simulink model "M004_refor_control"  (R2021a)
settings: Solver=VariableStepAuto  StartTime=0.0  StopTime=3  RelTol=1e-3
values from neighbouring files (symbols this model uses):
  MM = struct2array(MM)    [M004_init_refor_meca.m]
undefined symbols (not defined in the file or in its folder): params
settings Model: Creator=djoroya  LastModifiedBy=djoroya

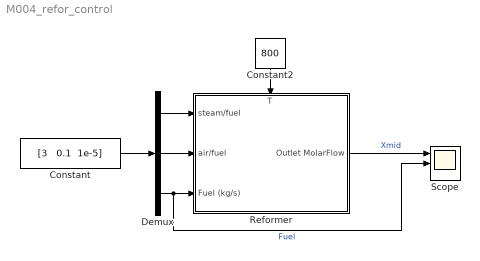
== system M004_refor_control ==
  Constant : Constant  Value="[3   0.1  1e-5]"
  Constant2 : Constant  Value=800
  Demux : Demux  Outputs=3
  Reformer : Subsystem
      settings: PortSchema="{\"entries\":[{\"content\":{\"sides\":[{\"content\":{\"connectorIds\":[\"In1\",\"In2\",\"In3\"]},\"type\":\"ConnectorPlacement.EquallySpacedRectSide\",\"uuid\":\"bba98e9a-4a8f-433d-80b6-6443373beb37\"},{\"content\":{\"connectorIds\":[\"Out1\"],\"side\":\"RIGHT\"},\"type\":\"ConnectorPlacement.EquallySpacedRectSide\",\"uuid\":\"bb8208fa-3ad6-4550-bb87-9c458da504c5\"},{\"content\":{\"connectorIds\":[\"In4\"],\"side\":\"TOP\"},\"type\":\"ConnectorPlacement.EquallySpacedRectSide\",\"uuid\":\"10760c79-2681-4834-b090-bc5e1ffe83d8\"}]},\"type\":\"ConnectorPlacement.EquallySpacedConnector\",\"uuid\":\"c7bbf7d3-64d5-4f0e-88ff-bb50ba74e7ab\"}],\"packageUris\":[\"http://schema.mathworks.com/mf0/Connector/R2020b\"],\"version\":\"1.0\"}"
  Scope : Scope  NumInputPorts=3
  wires:
  Reformer/1(Outlet MolarFlow) -> Scope/1  "Xmid"
  Constant2/1 -> Reformer/4(T)
  Constant/1 -> Demux/1
  Demux/2 -> Reformer/2(air/fuel)
  Demux/3 -> Scope/2, Reformer/3(Fuel (kg/s))  "Fuel"
  Demux/1 -> Reformer/1(steam/fuel)

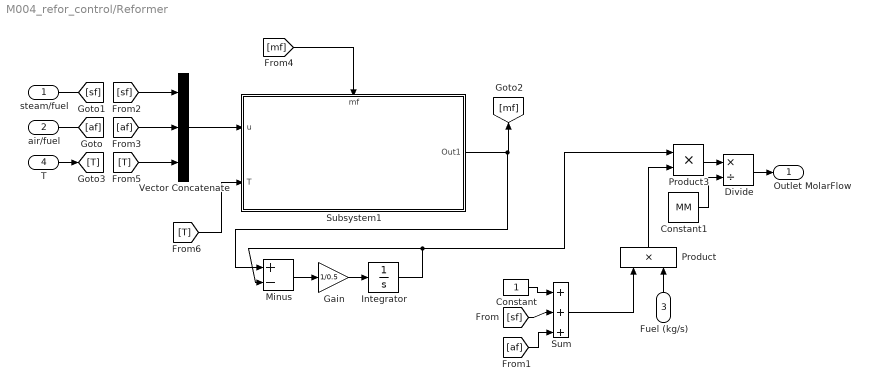
== system M004_refor_control/Reformer ==
  steam/fuel : Inport
  air/fuel : Inport  Port=2
  Fuel (kg/s) : Inport  Port=3
  T : Inport  Port=4
  Constant : Constant
  Constant1 : Constant  Value=MM
  Divide : Product  Inputs=*/
  Gain : Gain  Gain=1/0.5
  Integrator : Integrator
  Minus : Sum  Inputs=+-
  Product : Product
  Product3 : Product
  Subsystem1 : Subsystem
      settings: PortSchema="{\"entries\":[{\"content\":{\"sides\":[{\"content\":{\"connectorIds\":[\"In1\",\"In2\"]},\"type\":\"ConnectorPlacement.EquallySpacedRectSide\",\"uuid\":\"d4e99106-98ee-451f-9de6-7a659962116b\"},{\"content\":{\"connectorIds\":[\"Out1\"],\"side\":\"RIGHT\"},\"type\":\"ConnectorPlacement.EquallySpacedRectSide\",\"uuid\":\"1c23e47e-8482-4a31-825f-a97525afd909\"},{\"content\":{\"connectorIds\":[\"In3\"],\"side\":\"TOP\"},\"type\":\"ConnectorPlacement.EquallySpacedRectSide\",\"uuid\":\"6970ef93-3b6d-46bc-9d04-0338d9ef962f\"}]},\"type\":\"ConnectorPlacement.EquallySpacedConnector\",\"uuid\":\"3dd46f6e-571c-473b-b07f-3e0a0086d241\"}],\"packageUris\":[\"http://schema.mathworks.com/mf0/Connector/R2020b\"],\"version\":\"1.0\"}"
  Sum : Sum  Inputs=|+++
  Vector Concatenate : Concatenate  NumInputs=3
  Outlet MolarFlow : Outport
  wires:
  [af] -> Vector Concatenate/2
  [sf] -> Vector Concatenate/1
  [sf] -> Sum/2
  steam/fuel/1 -> [sf]
  Product/1 -> Product3/2
  air/fuel/1 -> [af]
  [af] -> Sum/3
  Constant/1 -> Sum/1
  Fuel (kg/s)/1 -> Product/2
  Sum/1 -> Product/1
  T/1 -> [T]
  [T] -> Vector Concatenate/3
  Subsystem1/1(Out1) -> [mf], Minus/1
  Vector Concatenate/1 -> Subsystem1/1(u)
  [mf] -> Subsystem1/3(mf)
  [T] -> Subsystem1/2(T)
  Integrator/1 -> Product3/1, Minus/2
  Minus/1 -> Gain/1
  Gain/1 -> Integrator/1
  Product3/1 -> Divide/1
  Divide/1 -> Outlet MolarFlow/1
  Constant1/1 -> Divide/2

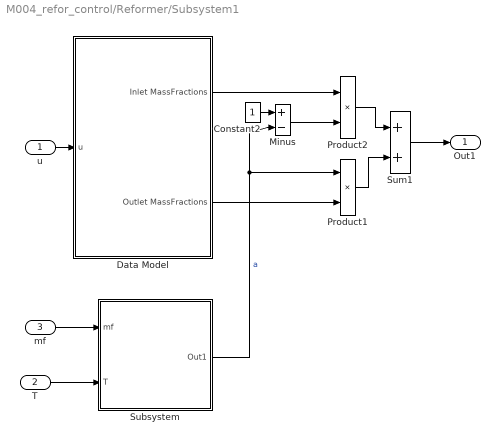
== system M004_refor_control/Reformer/Subsystem1 ==
  u : Inport
  T : Inport  Port=2
  mf : Inport  Port=3
  Constant2 : Constant
  Data Model : Subsystem
  Minus : Sum  Inputs=+-
  Product1 : Product
  Product2 : Product
  Subsystem : Subsystem
  Sum1 : Sum  Inputs=|++
  Out1 : Outport
  wires:
  Data Model/1(Inlet MassFractions) -> Product2/1
  Sum1/1 -> Out1/1
  Subsystem/1(Out1) -> Minus/2, Product1/1  "a"
  mf/1 -> Subsystem/1(mf)
  Constant2/1 -> Minus/1
  Product2/1 -> Sum1/1
  u/1 -> Data Model/1(u)
  T/1 -> Subsystem/2(T)
  Data Model/2(Outlet MassFractions) -> Product1/2
  Minus/1 -> Product2/2
  Product1/1 -> Sum1/2

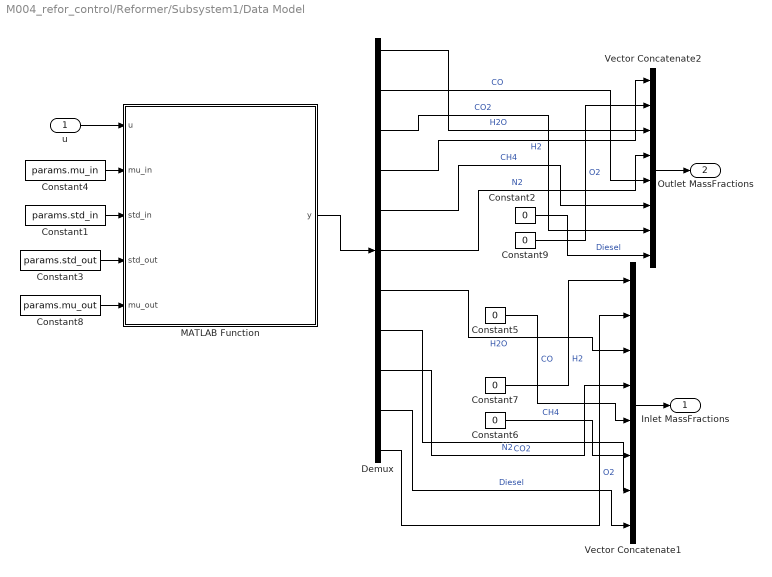
== system M004_refor_control/Reformer/Subsystem1/Data Model ==
  u : Inport
  Constant1 : Constant  Value=params.std_in
  Constant{2,5..7,9} (5 alike) : Constant  Value=0
  Constant3 : Constant  Value=params.std_out
  Constant4 : Constant  Value=params.mu_in
  Constant8 : Constant  Value=params.mu_out
  Demux : Demux  Outputs=11
  MATLAB Function : MATLAB Function  TreatAsAtomicUnit=on
  Vector Concatenate1 : Concatenate  NumInputs=8
  Vector Concatenate2 : Concatenate  NumInputs=8
  Inlet MassFractions : Outport
  Outlet MassFractions : Outport  Port=2
  wires:
  Vector Concatenate1/1 -> Inlet MassFractions/1
  Constant6/1 -> Vector Concatenate1/6  "CH4"
  Demux/4 -> Vector Concatenate2/1  "H2"
  Demux/1 -> Vector Concatenate2/3  "H2O"
  Demux/2 -> Vector Concatenate2/5  "CO"
  Vector Concatenate2/1 -> Outlet MassFractions/1
  Constant5/1 -> Vector Concatenate1/5  "CO"
  Demux/5 -> Vector Concatenate2/6  "CH4"
  Constant4/1 -> MATLAB Function/2(mu_in)
  u/1 -> MATLAB Function/1(u)
  Constant1/1 -> MATLAB Function/3(std_in)
  Constant3/1 -> MATLAB Function/4(std_out)
  Constant8/1 -> MATLAB Function/5(mu_out)
  Demux/3 -> Vector Concatenate2/7  "CO2"
  MATLAB Function/1(y) -> Demux/1
  Demux/6 -> Vector Concatenate2/4  "N2"
  Demux/7 -> Vector Concatenate1/3  "H2O"
  Constant2/1 -> Vector Concatenate2/8  "Diesel"
  Demux/8 -> Vector Concatenate1/7  "CO2"
  Demux/9 -> Vector Concatenate1/4  "N2"
  Demux/10 -> Vector Concatenate1/8  "Diesel"
  Constant7/1 -> Vector Concatenate1/1  "H2"
  Demux/11 -> Vector Concatenate1/2  "O2"
  Constant9/1 -> Vector Concatenate2/2  "O2"

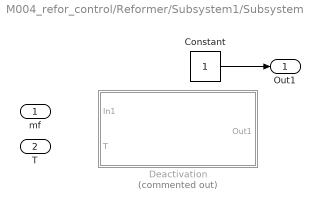
== system M004_refor_control/Reformer/Subsystem1/Subsystem ==
  mf : Inport
  T : Inport  Port=2
  Constant : Constant
  Deactivation : Subsystem  Commented=on  mask{k0=0.024, k=[0 0 0 0 0 0 0 ]', nd=1, Kw_ast=0, Ew=0}
  Out1 : Outport
  wires:
  Constant/1 -> Out1/1

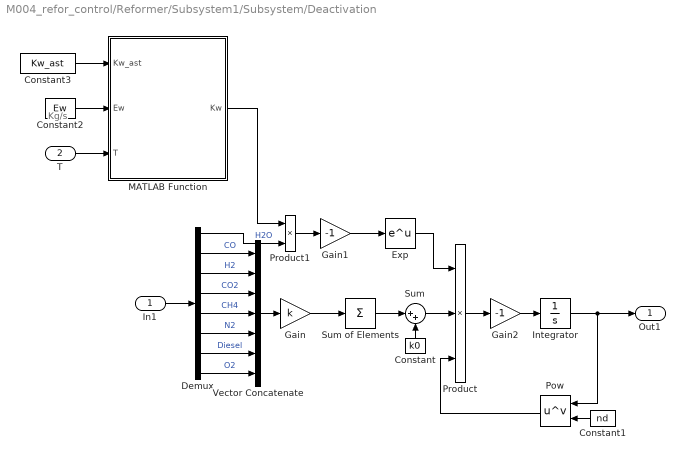
== system M004_refor_control/Reformer/Subsystem1/Subsystem/Deactivation ==
  note: Kg/s
  In1 : Inport
  T : Inport  Port=2
  Constant : Constant  Value=k0
  Constant1 : Constant  Value=nd
  Constant2 : Constant  Value=Ew
  Constant3 : Constant  Value=Kw_ast
  Demux : Demux  Outputs=8
  Exp : Math  SaturateOnIntegerOverflow=on
  Gain : Gain  Gain=k
  Gain1 : Gain  Gain=-1
  Gain2 : Gain  Gain=-1
  Integrator : Integrator  InitialCondition=1
  MATLAB Function : MATLAB Function  TreatAsAtomicUnit=on
  Pow : Math  Operator=pow  RndMeth=Zero  SaturateOnIntegerOverflow=on
  Product : Product  Inputs=3
  Product1 : Product
  Sum : Sum  Inputs=|++
  Sum of Elements : Sum  Inputs=+
  Vector Concatenate : Concatenate  NumInputs=7
  Out1 : Outport
  wires:
  Integrator/1 -> Out1/1, Pow/1
  In1/1 -> Demux/1
  Demux/6 -> Vector Concatenate/5  "N2"
  Demux/5 -> Vector Concatenate/4  "CH4"
  Demux/4 -> Vector Concatenate/3  "CO2"
  Demux/3 -> Vector Concatenate/2  "H2"
  Demux/2 -> Vector Concatenate/1  "CO"
  Vector Concatenate/1 -> Gain/1
  Constant/1 -> Sum/2
  Sum/1 -> Product/2
  Demux/1 -> Product1/2  "H2O"
  Exp/1 -> Product/1
  Pow/1 -> Product/3
  Constant1/1 -> Pow/2
  Gain/1 -> Sum of Elements/1
  Sum of Elements/1 -> Sum/1
  Product/1 -> Gain2/1
  Gain2/1 -> Integrator/1
  Demux/7 -> Vector Concatenate/6  "Diesel"
  T/1 -> MATLAB Function/3(T)
  Constant2/1 -> MATLAB Function/2(Ew)
  Constant3/1 -> MATLAB Function/1(Kw_ast)
  MATLAB Function/1(Kw) -> Product1/1
  Product1/1 -> Gain1/1
  Gain1/1 -> Exp/1
  Demux/8 -> Vector Concatenate/7  "O2"

== matlab function M004_refor_control/Reformer/Subsystem1/Data Model/MATLAB Function ==
  data: u input; y output; mu_in input; std_in input; std_out input; mu_out input
function y = fcn(u,mu_in,std_in,std_out,mu_out)

y = REFORMER_mf((u - mu_in)./std_in).*std_out + mu_out;

== matlab function M004_refor_control/Reformer/Subsystem1/Subsystem/Deactivation/MATLAB Function ==
  data: Kw_ast input; Kw output; Ew input; T input
function Kw = fcn(Kw_ast,Ew,T)

R = 8.314472;% J/(mol K) 

Kw = Kw_ast*exp(-Ew/R*(1/(T+273.15) - 1/573));
